simulink model "CGMRES"  (R2015a)
settings: Solver=ode45  StartTime=0.0  StopTime=tsim  RelTol=1e-3
values from neighbouring files (symbols this model uses):
  dSamplingPeriod = 0.001    [CGMRES_config.m]
  Ig = 0.0125    [CGMRES_config.m]
  M = 0.894    [CGMRES_config.m]
  r = 0.0485    [CGMRES_config.m]
undefined symbols (not defined in the file or in its folder): cgmres, sys
settings Model: Creator=hamada  LastModifiedBy=hamada

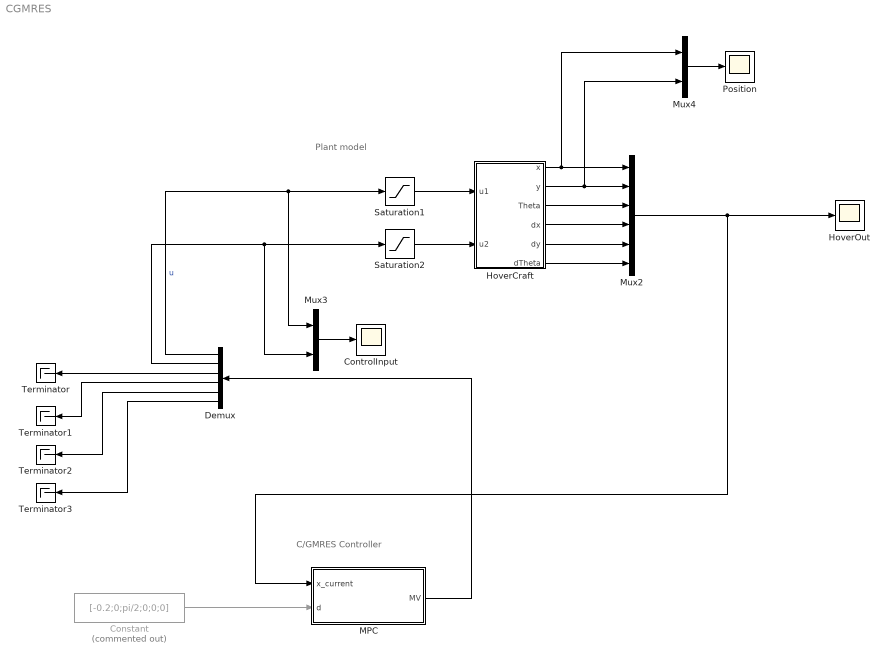
== system CGMRES ==
  note: C/GMRES Controller
  note: Plant model
  Constant : Constant  Commented=on  Value=[-0.2;0;pi/2;0;0;0]
  ControlInput : Scope
      settings: YMin=-0.125  YMax=0.35  SaveName=Output1  SampleInput=on  SampleTime=0.01
  Demux : Demux  Outputs=6
  HoverCraft : Subsystem
  HoverOut : Scope
      settings: YMin=-2.25  YMax=0.5  SaveName=HoverOut  SampleInput=on  SampleTime=0.01
  MPC : MATLAB Function  TreatAsAtomicUnit=on  SystemSampleTime=dSamplingPeriod
  Mux2 : Mux  Inputs=6
  Mux3 : Mux  Inputs=2
  Mux4 : Mux  Inputs=2
  Position : Scope
      settings: TimeRange=20  YMin=-6  YMax=0.5  SaveName=Output2  SampleInput=on  SampleTime=0.01
  Saturation1 : Saturate  UpperLimit=0.342  LowerLimit=-0.121
  Saturation2 : Saturate  UpperLimit=0.342  LowerLimit=-0.121
  Terminator{,1..3} (4 alike) : Terminator
  wires:
  Demux/1 -> Mux3/1, Saturation1/1  "u"
  MPC/1(MV) -> Demux/1
  Demux/3 -> Terminator/1
  Demux/4 -> Terminator1/1
  Demux/2 -> Mux3/2, Saturation2/1
  HoverCraft/1(x) -> Mux4/1, Mux2/1
  HoverCraft/2(y) -> Mux4/2, Mux2/2
  HoverCraft/3(Theta) -> Mux2/3
  Saturation1/1 -> HoverCraft/1(u1)
  Saturation2/1 -> HoverCraft/2(u2)
  HoverCraft/6(dTheta) -> Mux2/6
  HoverCraft/5(dy) -> Mux2/5
  HoverCraft/4(dx) -> Mux2/4
  Demux/5 -> Terminator2/1
  Demux/6 -> Terminator3/1
  Mux3/1 -> ControlInput/1
  Mux4/1 -> Position/1
  Constant/1 -> MPC/2(d)
  Mux2/1 -> MPC/1(x_current), HoverOut/1

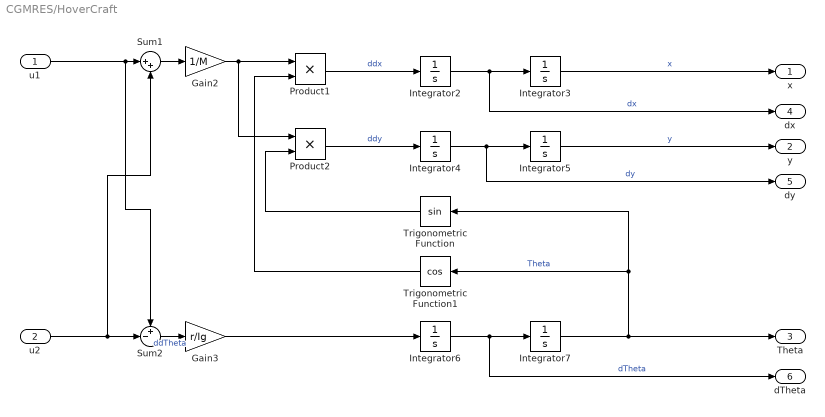
== system CGMRES/HoverCraft ==
  u1 : Inport
  u2 : Inport  Port=2
  Gain2 : Gain  Gain=1/M
  Gain3 : Gain  Gain=r/Ig
  Integrator2 : Integrator  InitialCondition=sys.x0(4)
  Integrator3 : Integrator  InitialCondition=sys.x0(1)
  Integrator4 : Integrator  InitialCondition=sys.x0(5)
  Integrator5 : Integrator  InitialCondition=sys.x0(2)
  Integrator6 : Integrator  InitialCondition=sys.x0(6)
  Integrator7 : Integrator  InitialCondition=sys.x0(3)
  Product1 : Product
  Product2 : Product
  Sum1 : Sum  Inputs=|++
  Sum2 : Sum  Inputs=+-|
  Trigonometric Function : Trigonometry
  Trigonometric Function1 : Trigonometry  Operator=cos
  x : Outport
  y : Outport  Port=2
  Theta : Outport  Port=3
  dx : Outport  Port=4
  dy : Outport  Port=5
  dTheta : Outport  Port=6
  wires:
  Gain3/1 -> Integrator6/1
  Gain2/1 -> Product2/1, Product1/1
  u1/1 -> Sum2/1, Sum1/1
  Trigonometric Function1/1 -> Product1/2
  u2/1 -> Sum2/2, Sum1/2
  Product1/1 -> Integrator2/1  "ddx"
  Integrator4/1 -> dy/1, Integrator5/1  "dy"
  Integrator6/1 -> dTheta/1, Integrator7/1  "dTheta"
  Sum2/1 -> Gain3/1  "ddTheta"
  Sum1/1 -> Gain2/1
  Integrator5/1 -> y/1  "y"
  Product2/1 -> Integrator4/1  "ddy"
  Integrator2/1 -> dx/1, Integrator3/1  "dx"
  Integrator3/1 -> x/1  "x"
  Integrator7/1 -> Trigonometric Function/1, Trigonometric Function1/1, Theta/1  "Theta"
  Trigonometric Function/1 -> Product2/2

== matlab function CGMRES/MPC ==
  data: x_current input size=6; d input size=6; sys parameter; cgmres parameter; MV output size=6; dSamplingPeriod parameter size=1
function MV = MPC( x_current, d, sys, cgmres, dSamplingPeriod )
    %#codegen
    persistent flag; % 初回フラグ
    persistent du; % 操作量の変化量（前回値）
    persistent u; % 操作量（前回値）
    persistent T; % 予測区間
    
    if ( isempty( flag ) )
        flag = 0;
    end
    
    if ( isempty( du ) )
        du = zeros( cgmres.len_u * cgmres.dv, 1 );
    end
    
    if ( isempty( u ) )
        u = zeros( cgmres.len_u * cgmres.dv, 1 );
    end
    
    if ( isempty( T ) )
        T = 0;
    end
    
    % 初回のみ操作量の計算方法が異なる
    if ( 0 == flag )
        du = repmat( cgmres.u0, cgmres.dv, 1 );
        u = du;
        flag = 1;
    end 
    
    MV = u(1:cgmres.len_u);
    
    % du = rand( size( du ) ); % 操作量の変化量の初期値は任意に選べるが，前回値を利用すると収束が速い
    du = GMRES( x_current, du, u, d, T, sys, cgmres );
    u = u + du * dSamplingPeriod;
    
    T = cgmres.T_outGain * T + cgmres.T_inGain;
end
